simulink model "vy_estimator_base"  (R2024b)
settings: Solver=FixedStepAuto  StartTime=0.0  StopTime=10.0  RelTol=1e-3
undefined symbols (not defined in the file): Discrete, LM, Time
libraries: simulink_extras x1, ctrlSharedLib x1
settings Model: Creator=lukec  LastModifiedBy=lukec
settings OptimizationCC: DefaultParameterBehavior=Inlined  EnhancedBackFolding=on  PassReuseOutputArgsAs=Individual arguments  ZeroExternalMemoryAtStartup=off  ZeroInternalMemoryAtStartup=off  OptimizeBlockOrder=speed  DifferentSizesBufferReuse=on  OptimizationCustomize=off  EfficientTunableParamExpr=on
settings DebuggingCC: ParameterTunabilityLossMsg=error
settings HardwareCC: ProdBitPerPointer=32  ProdBitPerSizeT=32  ProdBitPerPtrDiffT=32  ProdLargestAtomicInteger=Long  ProdLargestAtomicFloat=Double  ProdWordSize=32  ProdHWDeviceType=ARM Compatible->ARM Cortex-M
settings SFSimCC: MATLABDynamicMemAlloc=off
settings RTWCC: Description=Embedded Coder  SystemTargetFile=ert.tlc  GenCodeOnly=on  PackageGeneratedCodeAndArtifacts=on  TemplateMakefile=ert_default_tmf  Toolchain=CMake  TargetLang=C++  HalideCodeGeneration=on
settings CodeAppCC: ForceParamTrailComments=on  IgnoreCustomStorageClasses=off  MaxIdLength=255  OperatorAnnotations=on  SimulinkDataObjDesc=on  SFDataObjDesc=on  InsertBlockDesc=on
settings ERTTargetCC: TargetLangStandard=C++17 (ISO)  CodeInterfacePackaging=C++ class  RootIOFormat=Structure reference  ERTCustomFileTemplate=example_file_process.tlc  ArrayContainerType=std::array

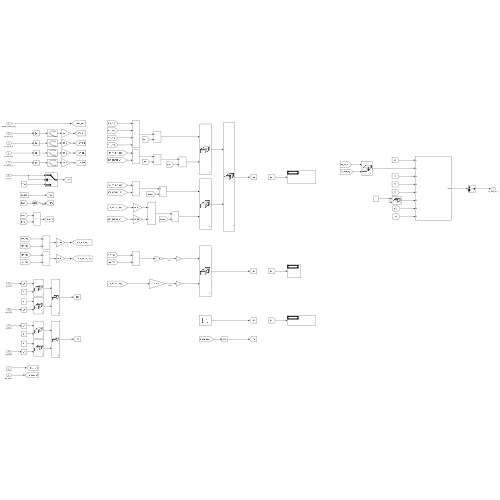
[thumbnail: Simulink's stored preview of the top-level diagram]
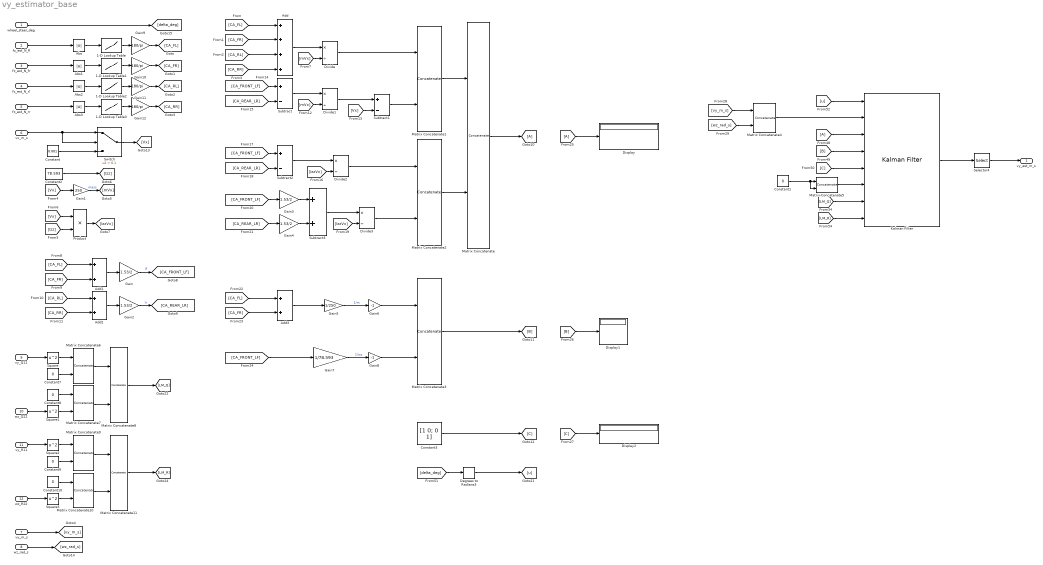
== system vy_estimator_base ==
  wheel_steer_deg : Inport  PortDimensions=1
  fz_est_N_fl : Inport  Port=2
  fz_est_N_fr : Inport  Port=3
  fz_est_N_rl : Inport  Port=4
  fz_est_N_rr : Inport  Port=5
  vx_m_s : Inport  Port=6
  vy_m_s : Inport  Port=7
  wz_rad_s : Inport  Port=8
  vy_Q11 : Inport  Port=9
  wz_Q22 : Inport  Port=10
  vy_R11 : Inport  Port=11
  wz_R22 : Inport  Port=12
  1-D Lookup Table{,1..3} (4 alike) : Lookup_n-D  NumberOfTableDimensions=1  BreakpointsForDimension1=LM.FZtest * -1  Table=LM.CA  ExtrapMethod=Clip  UseLastTableValue=on  InternalRulePriority=Speed  RndMeth=Simplest
  Abs{,1..3} (4 alike) : Abs  SaturateOnIntegerOverflow=off
  Add : Sum  Inputs=++++
  Add1 : Sum
  Add2 : Sum
  Add3 : Sum
  Constant : Constant  Value=0.001
  Constant{1,7..10} (5 alike) : Constant  Value=0
  Constant2 : Constant  Value=78.593
  Constant3 : Constant  Value=[1 0; 0 1]
  Degrees to Radians3 : simulink_extras/Transformations/Degrees to Radians
  Display : Display
  Display1 : Display
  Display2 : Display
  Divide{,1..3} (4 alike) : Product  Inputs=*/
  From25 : From
  From48 : From
  Gain{,2..4} (4 alike) : Gain  Gain=1.53/2
  Gain1 : Gain  Gain=250
  Gain{9..12} (4 alike) : Gain  Gain=180/pi
  Gain5 : Gain  Gain=1/250
  Gain6 : Gain  Gain=-1
  Gain7 : Gain  Gain=1/78.593
  Gain8 : Gain  Gain=-1
  Goto10 : Goto
  Kalman Filter : ctrlSharedLib/Kalman Filter  TimeDomain=Discrete-Time  UseCurrentEstimator=on  ModelSource=Input port  ModelSourceVariable=ss(0.95,1,1,0,1)  A=0.95  B=1  C=1  D=0  NumberOfStates=2  NumberOfInputs=1  NumberOfOutputs=2  InitialEstimateSource=Dialog  X0=0  P0=10  UseK=off  UseGH=off  NumberOfProcessNoiseInputs=1  G=1  TimeInvariantG=on  H=0  TimeInvariantH=on  Q=diag([5^2 1^2])  TimeInvariantQ=off  R=diag([0.1^2 0.01^2])  TimeInvariantR=off  N=0  TimeInvariantN=on  AddInputPort=on  AddEnablePort=off  OutputEstimatedY=off  OutputP=off  Ts=0.004
  Matrix Concatenate{,3..7,9..10} (8 alike) : Concatenate  Mode=Multidimensional array
  Matrix Concatenate{1..2,8,11} (4 alike) : Concatenate  Mode=Multidimensional array  ConcatenateDimension=2
  Product : Product
  Selector4 : Selector  InputPortWidth=2  IndexOptions=Index vector (dialog)  Indices=1  OutputSizes=1
  Square{,1..3} (4 alike) : Math  Operator=square
  Subtract : Sum  Inputs=+-
  Subtract1 : Sum  Inputs=+-
  Subtract2 : Sum  Inputs=+-
  Subtract3 : Sum
  Switch : Switch  Criteria=u2 > Threshold  Threshold=0.1  SaturateOnIntegerOverflow=off  InputSameDT=off
  vy_est_m_s : Outport
  wires:
  fz_est_N_rr/1 -> Abs3/1
  [IzzVx] -> Divide2/2
  [CA_RL] -> Add/3
  wheel_steer_deg/1 -> [delta_deg]
  [B] -> Kalman Filter/4
  Abs2/1 -> 1-D Lookup Table2/1
  Add1/1 -> Gain/1
  Gain/1 -> [CA_FRONT_LF]  "lf"
  [CA_RR] -> Add2/2
  Matrix Concatenate2/1 -> Matrix Concatenate/2
  [u] -> Kalman Filter/1
  Abs3/1 -> 1-D Lookup Table3/1
  [CA_FL] -> Add/1
  Subtract1/1 -> Matrix Concatenate1/2
  Gain4/1 -> Subtract3/2
  [Izz] -> Product/2
  Gain8/1 -> Matrix Concatenate3/2
  Matrix Concatenate4/1 -> Kalman Filter/2
  [B] -> Display1/1
  [CA_FRONT_LF] -> Subtract/1
  vx_m_s/1 -> Switch/1, Switch/2
  Kalman Filter/1 -> Selector4/1
  Add3/1 -> Gain5/1
  Matrix Concatenate5/1 -> Kalman Filter/6
  1-D Lookup Table1/1 -> Gain10/1
  [Vx] -> Product/1
  [CA_FR] -> Add/2
  Divide2/1 -> Matrix Concatenate2/1
  Divide1/1 -> Subtract1/1
  [CA_FR] -> Add1/2
  Gain11/1 -> [CA_RL]
  Gain6/1 -> Matrix Concatenate3/1
  Subtract/1 -> Divide1/1
  Matrix Concatenate/1 -> Goto10/1
  [CA_RL] -> Add2/1
  [CA_FL] -> Add3/1
  1-D Lookup Table3/1 -> Gain12/1
  [CA_REAR_LR] -> Subtract2/2
  Divide3/1 -> Matrix Concatenate2/2
  From48/1 -> Kalman Filter/3
  Selector4/1 -> vy_est_m_s/1
  Switch/1 -> [Vx]
  fz_est_N_fl/1 -> Abs/1
  Add/1 -> Divide/1
  Divide/1 -> Matrix Concatenate1/1
  Product/1 -> [IzzVx]
  Constant/1 -> Switch/3
  fz_est_N_fr/1 -> Abs1/1
  Gain2/1 -> [CA_REAR_LR]  "lr"
  [CA_REAR_LR] -> Subtract/2
  Subtract3/1 -> Divide3/1
  Add2/1 -> Gain2/1
  Gain3/1 -> Subtract3/1
  [C] -> Display2/1
  [delta_deg] -> Degrees to Radians3/1
  [IzzVx] -> Divide3/2
  Gain12/1 -> [CA_RR]
  Gain5/1 -> Gain6/1  "1/m"
  Gain7/1 -> Gain8/1  "1/Izz"
  Subtract2/1 -> Divide2/1
  [CA_FRONT_LF] -> Gain3/1
  Gain10/1 -> [CA_FR]
  [CA_FRONT_LF] -> Gain7/1
  Abs1/1 -> 1-D Lookup Table1/1
  [CA_REAR_LR] -> Gain4/1
  [mVx] -> Divide1/2
  From25/1 -> Display/1
  [CA_FR] -> Add3/2
  Matrix Concatenate3/1 -> [B]
  [Vx] -> Subtract1/2
  fz_est_N_rl/1 -> Abs2/1
  1-D Lookup Table2/1 -> Gain11/1
  Abs/1 -> 1-D Lookup Table/1
  Gain9/1 -> [CA_FL]
  [mVx] -> Divide/2
  Constant1/1 -> Matrix Concatenate5/1, Matrix Concatenate5/2
  Degrees to Radians3/1 -> [u]
  [CA_FL] -> Add1/1
  [CA_FRONT_LF] -> Subtract2/1
  Constant3/1 -> [C]
  [C] -> Kalman Filter/5
  Matrix Concatenate1/1 -> Matrix Concatenate/1
  [CA_RR] -> Add/4
  Constant2/1 -> [Izz]
  1-D Lookup Table/1 -> Gain9/1
  [Vx] -> Gain1/1
  Gain1/1 -> [mVx]  "mass"
  vy_Q11/1 -> Square/1
  wz_Q22/1 -> Square1/1
  Square/1 -> Matrix Concatenate6/1
  Constant7/1 -> Matrix Concatenate6/2
  Matrix Concatenate6/1 -> Matrix Concatenate8/1
  Square1/1 -> Matrix Concatenate7/2
  Constant8/1 -> Matrix Concatenate7/1
  Matrix Concatenate7/1 -> Matrix Concatenate8/2
  Matrix Concatenate8/1 -> [LM_Q]
  Matrix Concatenate11/1 -> [LM_R]
  Matrix Concatenate10/1 -> Matrix Concatenate11/2
  Constant10/1 -> Matrix Concatenate10/1
  Square3/1 -> Matrix Concatenate10/2
  Matrix Concatenate9/1 -> Matrix Concatenate11/1
  Constant9/1 -> Matrix Concatenate9/2
  Square2/1 -> Matrix Concatenate9/1
  wz_R22/1 -> Square3/1
  vy_R11/1 -> Square2/1
  [LM_Q] -> Kalman Filter/7
  [LM_R] -> Kalman Filter/8
  vy_m_s/1 -> [vy_m_s]
  [vy_m_s] -> Matrix Concatenate4/1
  wz_rad_s/1 -> [wz_rad_s]
  [wz_rad_s] -> Matrix Concatenate4/2
